simulink model "CCCV_Charging"  (R2024b)
settings: Solver=VariableStepAuto  StartTime=0.0  StopTime=100  RelTol=1e-3
undefined symbols (not defined in the file): Ion, Lithium
libraries: spsIdealSwitchLib x2, spsBatteryLib x1, spsControlledCurrentSourceLib x1, spsDCVoltageSourceLib x1, spsDiodeLib x1, spsSeriesRLCBranchLib x1, sps_lib x1
settings Model: Creator=yeswa  LastModifiedBy=yeswa
settings DebuggingCC: AlgebraicLoopMsg=none

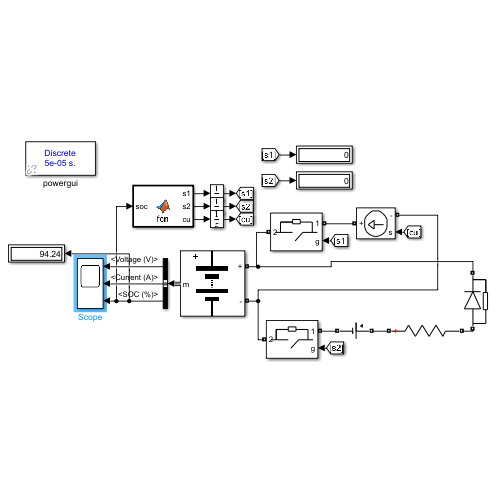
[thumbnail: Simulink's stored preview of the top-level diagram]
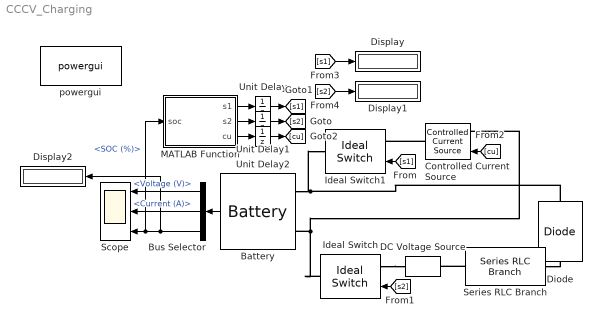
== system CCCV_Charging ==
  Battery : spsBatteryLib/Battery  BatType=Lithium-Ion  NomV=3.7  NomQ=5.4  SOC=78  Batt_Tr=30  PresetModel=on  MaxQ=5.4  MinV=2.775  FullV=4.3068  Dis_rate=2.3478  R=0.0068519  Normal_OP=4.8835  expZone="[3.9974      0.2653]"
  Bus Selector : BusSelector  OutputSignals=Voltage (V),Current (A),SOC (%)
  Controlled Current Source : spsControlledCurrentSourceLib/Controlled Current Source  Initialize=on  Source_Type=DC  Amplitude=2  Phase=0  Frequency=0  Measurements=None
  DC Voltage Source : spsDCVoltageSourceLib/DC Voltage Source  Amplitude=100  Measurements=None
  Diode : spsDiodeLib/Diode  Ron=0.001  Lon=0  Vf=0.8  IC=0  UseSnubber=0  Rs=500  Cs=250e-9  Measurements=off
  Display : Display
  Display1 : Display
  Display2 : Display
  Ideal Switch : spsIdealSwitchLib/Ideal Switch  Ron=0.001  Lon=0  IC=0  Rs=1e5  Cs=inf  Measurements=off
  Ideal Switch1 : spsIdealSwitchLib/Ideal Switch  Ron=0.001  Lon=0  IC=0  Rs=1e5  Cs=inf  Measurements=off
  MATLAB Function : MATLAB Function  TreatAsAtomicUnit=on
  Scope : Scope  NumInputPorts=3
  Series RLC Branch : spsSeriesRLCBranchLib/Series RLC Branch  LConnTagsString=__new0  RConnTagsString=__new0  BranchType=R  Resistance=1  Inductance=1e-3  SetiL0=off  InitialCurrent=0  Capacitance=1e-6  Setx0=off  InitialVoltage=0  Measurements=None
  Unit Delay : UnitDelay  SampleTime=5e-05  HasFrameUpgradeWarning=on
  Unit Delay1 : UnitDelay  SampleTime=5e-05  HasFrameUpgradeWarning=on
  Unit Delay2 : UnitDelay  SampleTime=5e-05  HasFrameUpgradeWarning=on
  powergui : sps_lib/powergui  Priority=1  SimulationMode=Discrete  SampleTime=5e-5  frequency=60  Iterations=50  frequencyindice=0  Pbase=100e6  ErrMax=1e-4  UnitsV=kV  UnitsW=MW  buscounter=0  FunctionMessages=off  echomessages=off  EnableUseOfTLC=off  CurrentSourceSwitches=off  DisableSnubberDevices=off  DisableRonSwitches=off  DisableVfSwitches=off  DisplayEquations=off  AutomaticDiscreteSolvers=off  SolverType=Tustin/Backward Euler (TBE)  Interpol=off  ExternalGateDelay=off  methode=off  Ts=100  x0status=blocks  SPID=on  SwTol=0  HookPort=off  NonlinearTolerance=1e-4  nMaxIteration=100  ContinueOnMaxIteration=off  RestoreLinks=warning  ResistiveCurrentMeasurement=off  Frange=[0:2:500]  Ylog=off  Xlog=on  ShowGrid=off  save=off  variable=ZData  structure=0  ZoomFFT=off  StartTime=0.0  cycles=1  DisplayStyle=1  fundamental=60  FreqAxis=off  MaxFrequency=1000  frequencyindicesteady=1  RmsSteady=1  display=off
  wires:
  Battery/1 -> Bus Selector/1
  Bus Selector/2 -> Scope/2  "<Current (A)>"
  Bus Selector/1 -> Scope/1  "<Voltage (V)>"
  Bus Selector/3 -> Display2/1, MATLAB Function/1(soc), Scope/3  "<SOC (%)>"
  [s1] -> Ideal Switch1/1
  [s2] -> Ideal Switch/1
  [cu] -> Controlled Current Source/1
  [s1] -> Display/1
  [s2] -> Display1/1
  MATLAB Function/1(s1) -> Unit Delay/1
  MATLAB Function/2(s2) -> Unit Delay1/1
  MATLAB Function/3(cu) -> Unit Delay2/1
  Unit Delay2/1 -> [cu]
  Unit Delay1/1 -> [s2]
  Unit Delay/1 -> [s1]
  connections:
  Ideal Switch/RConn1 -- Controlled Current Source/LConn1 -- Battery/LConn2
  Ideal Switch/LConn1 -- DC Voltage Source/LConn1
  Series RLC Branch/LConn1 -- DC Voltage Source/RConn1
  Controlled Current Source/RConn1 -- Ideal Switch1/LConn1
  Series RLC Branch/RConn1 -- Diode/LConn1
  Battery/LConn1 -- Ideal Switch1/RConn1 -- Diode/RConn1

== matlab function CCCV_Charging/MATLAB Function ==
  data: soc input; s1 output; s2 output; cu output
function [s1,s2,cu] = fcn(soc)

if soc >= 0 && soc <= 80
    s1 = 1;
    s2 = 0;
    cu = 100;

elseif soc > 80 && soc <= 90
    s1 = 0;
    s2 = 1;
    cu = 0;

else
    s1 = 0;
    s2 = 0;
    cu = 0;
end

end
